simulink model "ES229A_HwTqCorrln"  (R2013b)
settings: Solver=FixedStepDiscrete  SolverMode=SingleTasking  StartTime=0.0  StopTime=1  FixedStep=0.002  RelTol=1e-3
undefined symbols (not defined in the file): ARCHGLBPRM_100MILLISEC_SEC_F32, FLTINJ_HWTQCORRLN_HWTQIDPTSIG, HwTqCorrlnChACmnModCmpLpFilActvnThd, HwTqCorrlnChACmnModCmpLpFilOutpLim, HwTqCorrlnChAImdtCorrlnChkFailThd, HwTqCorrlnChAImdtCorrlnChkPassThd, HwTqCorrlnChAStabStClrFltThd, HwTqCorrlnChAStabStSetFltThd, HwTqCorrlnChATqSumMaxLim, HwTqCorrlnChATraSumClrFltThd, HwTqCorrlnChATraSumSetFltThd, HwTqCorrlnChBCmnModCmpLpFilActvnThd, HwTqCorrlnChBCmnModCmpLpFilOutpLim, HwTqCorrlnChBImdtCorrlnChkFailThd, HwTqCorrlnChBImdtCorrlnChkPassThd, HwTqCorrlnChBStabStClrFltThd, HwTqCorrlnChBStabStSetFltThd, HwTqCorrlnChBTqSumMaxLim, HwTqCorrlnChBTraSumClrFltThd, HwTqCorrlnChBTraSumSetFltThd, HwTqCorrlnMaxStallTqA, HwTqCorrlnMaxStallTqB, HwTqCorrlnMaxStallTqC, HwTqCorrlnMaxStallTqD, HWTQSCA_CNT_U08, NtcNr1, NtcSts1, PARAMETERBYTE_CNT_U08, sigbuilder_block, SigQlfr1, STABSTLPFILSTVARIDELTALIM_HWNWTMTR_F32
libraries: simulink x25, Fil x12, NxtrLim x10, NxtrAbslt x6, FixdToFloat x2, FloatToFixdWithRound x2, LnrIntrpn x2, NxtrNvM x2
(part 2 of 4)

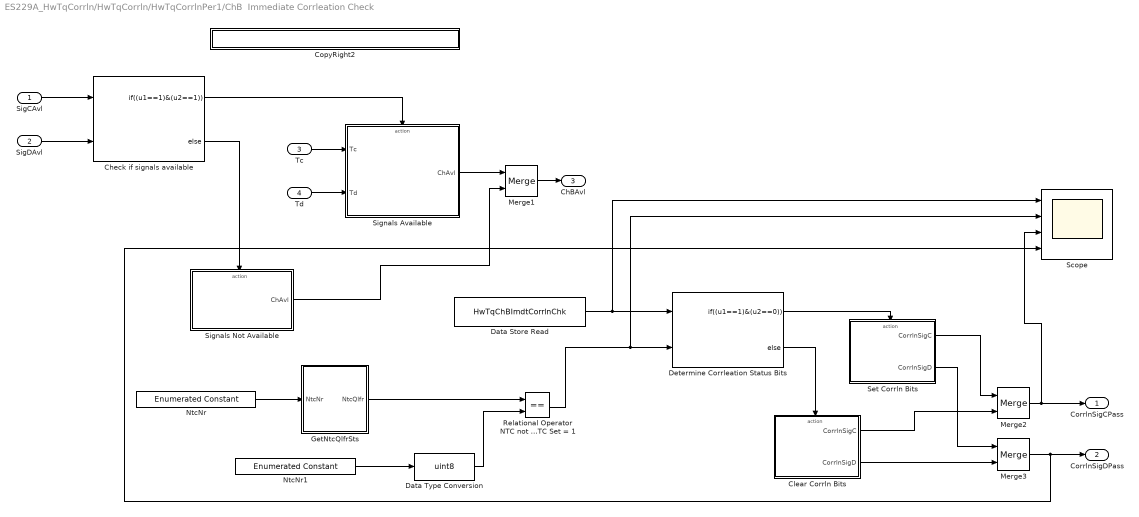
== system ES229A_HwTqCorrln/HwTqCorrln/HwTqCorrlnPer1/ChB  Immediate Corrleation Check ==
  SigCAvl : Inport
  SigDAvl : Inport  Port=2
  Tc : Inport  Port=3
  Td : Inport  Port=4
  Check if signals available : If  NumInputs=2  IfExpression=(u1==1)&(u2==1)
  Clear Corrln Bits : Subsystem  TreatAsAtomicUnit=on
  CopyRight2 : Subsystem  Description=|  mask(Copyright Information){none=on}
      | Copyright info block.                                               
      |                                                                     
      | Place copyright information at the top of every subsystem in design.
      mask prompts: none "No parameters"
      mask help: Place copyright information at the top of every subsystem in design.
      mask Display:
      | NxtrConf = 'Nexteer Confidential';
      | 
      | sys = bdroot; %handle for the current model ("system")
      | first = get_param(sys,'Created');
      | first = first(end-3:end);  %year is last four digits
      | 
      | last = get_param(sys,'LastModifiedDate');
      | if isempty(last)
      |     last = datestr(now,'yyyy');
      | else
      |     last = last(end-3:end);
      | end
      | 
      | if strcmp(first,last)
      |     fprintf('%s -- Copyright %s Nexteer',NxtrConf,first)
      | else
      |     fprintf('%s -- %s%s- %s Nexteer',NxtrConf,char(169),first,last)
      | end
  Data Store Read : DataStoreRead  DataStoreName=HwTqChBImdtCorrlnChk
  Data Type Conversion : DataTypeConversion  OutDataTypeStr=uint8
  Determine Corrleation Status Bits : If  NumInputs=2  IfExpression=(u1==1)&(u2==0)
  GetNtcQlfrSts : Subsystem  RequirementInfo={} %GIDa_b9216dd4_3d01_4ddd_95ef_a4798394f877  TreatAsAtomicUnit=on  mask(GetNTC){}
      mask help: GetNTC library block
      settings: RTWSystemCode=Inline
  Merge1 : Merge
  Merge2 : Merge
  Merge3 : Merge
  NtcNr : simulink/Sources/Enumerated Constant  OutDataTypeStr=Enum: NtcNr1  Value=NtcNr1.NTCNR_0X071  SampleTime=inf
  NtcNr1 : simulink/Sources/Enumerated Constant  OutDataTypeStr=Enum: SigQlfr1  Value=SigQlfr1.SIGQLFR_FAILD  SampleTime=inf
  "Relational Operator NTC not Set = 0, NTC Set = 1" : RelationalOperator  Operator===  OutDataTypeStr=boolean
  Scope : Scope  NumInputPorts=4
      settings: TimeRange=auto  MaxDataPoints=5000  SaveToWorkspace=off  SaveName=ScopeData8  YMin=-5~-5~-5~-5  YMax=5~5~5~5  SampleTime=-1
  Set Corrln Bits : Subsystem  TreatAsAtomicUnit=on
  Signals Available : Subsystem  RequirementInfo={'linktype_rmi_doors' '0000c477 (/ESG Group/FDD Module Requirements/EA4 Specific/ES229A_HwTqCorrln)' '#ES229A_114' 'true' 'REQ:ES229A_114' '' } %GIDa_b18ea54d_339b_4dd7_8965_346bd4b35b88  TreatAsAtomicUnit=on
  Signals Not Available : Subsystem  RequirementInfo={'linktype_rmi_doors' '0000c477 (/ESG Group/FDD Module Requirements/EA4 Specific/ES229A_HwTqCorrln)' '#ES229A_162' 'true' 'REQ:ES229A_162' '' } %GIDa_09088bdc_3033_45ea_8a6e_b545563978f2  TreatAsAtomicUnit=on
  CorrlnSigCPass : Outport
  CorrlnSigDPass : Outport  Port=2
  ChBAvl : Outport  Port=3
  wires:
  Tc/1 -> Signals Available/1(Tc)
  Td/1 -> Signals Available/2(Td)
  Merge3/1 -> Scope/4, CorrlnSigDPass/1
  Determine Corrleation Status Bits/2 -> Clear Corrln Bits/Action
  Determine Corrleation Status Bits/1 -> Set Corrln Bits/Action
  Set Corrln Bits/1(CorrlnSigC) -> Merge2/1
  Clear Corrln Bits/1(CorrlnSigC) -> Merge2/2
  Clear Corrln Bits/2(CorrlnSigD) -> Merge3/2
  NtcNr/1 -> GetNtcQlfrSts/1(NtcNr)
  Data Type Conversion/1 -> "Relational Operator NTC not Set = 0, NTC Set = 1"/2
  GetNtcQlfrSts/1(NtcQlfr) -> "Relational Operator NTC not Set = 0, NTC Set = 1"/1
  "Relational Operator NTC not Set = 0, NTC Set = 1"/1 -> Determine Corrleation Status Bits/2, Scope/2
  Check if signals available/1 -> Signals Available/Action
  Check if signals available/2 -> Signals Not Available/Action
  Data Store Read/1 -> Scope/1, Determine Corrleation Status Bits/1
  SigCAvl/1 -> Check if signals available/1
  SigDAvl/1 -> Check if signals available/2
  Merge2/1 -> Scope/3, CorrlnSigCPass/1
  Set Corrln Bits/2(CorrlnSigD) -> Merge3/1
  NtcNr1/1 -> Data Type Conversion/1
  Merge1/1 -> ChBAvl/1
  Signals Not Available/1(ChAvl) -> Merge1/2
  Signals Available/1(ChAvl) -> Merge1/1

== system ES229A_HwTqCorrln/HwTqCorrln/HwTqCorrlnPer1/CopyRight2 ==

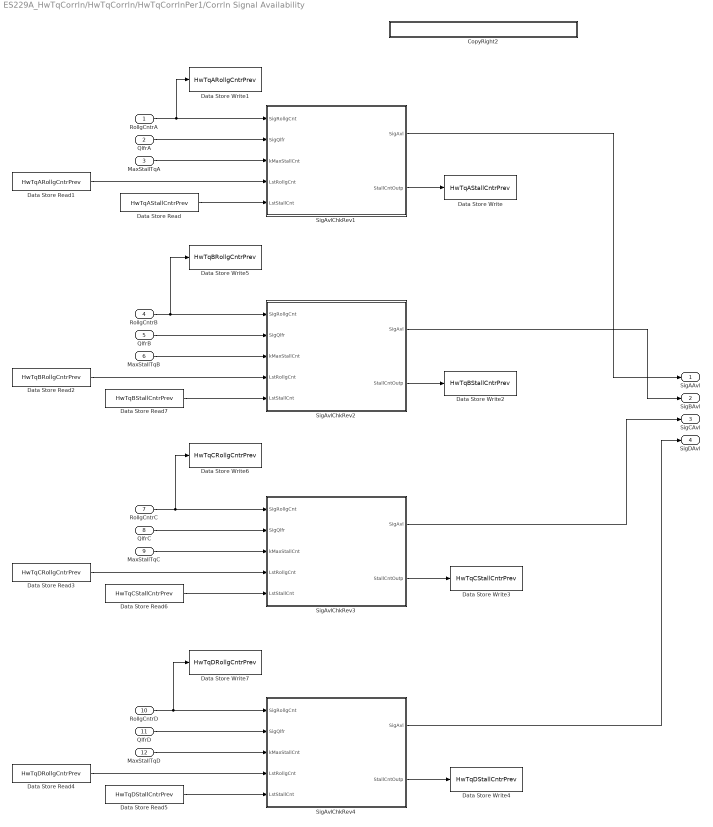
== system ES229A_HwTqCorrln/HwTqCorrln/HwTqCorrlnPer1/Corrln Signal Availability ==
  RollgCntrA : Inport
  QlfrA : Inport  Port=2
  MaxStallTqA : Inport  Port=3
  RollgCntrB : Inport  Port=4
  QlfrB : Inport  Port=5
  MaxStallTqB : Inport  Port=6
  RollgCntrC : Inport  Port=7
  QlfrC : Inport  Port=8
  MaxStallTqC : Inport  Port=9
  RollgCntrD : Inport  Port=10
  QlfrD : Inport  Port=11
  MaxStallTqD : Inport  Port=12
  CopyRight2 : Subsystem  Description=|  mask(Copyright Information){none=on}
      | Copyright info block.                                               
      |                                                                     
      | Place copyright information at the top of every subsystem in design.
      mask prompts: none "No parameters"
      mask help: Place copyright information at the top of every subsystem in design.
      mask Display:
      | NxtrConf = 'Nexteer Confidential';
      | 
      | sys = bdroot; %handle for the current model ("system")
      | first = get_param(sys,'Created');
      | first = first(end-3:end);  %year is last four digits
      | 
      | last = get_param(sys,'LastModifiedDate');
      | if isempty(last)
      |     last = datestr(now,'yyyy');
      | else
      |     last = last(end-3:end);
      | end
      | 
      | if strcmp(first,last)
      |     fprintf('%s -- Copyright %s Nexteer',NxtrConf,first)
      | else
      |     fprintf('%s -- %s%s- %s Nexteer',NxtrConf,char(169),first,last)
      | end
  Data Store Read : DataStoreRead  DataStoreName=HwTqAStallCntrPrev
  Data Store Read1 : DataStoreRead  DataStoreName=HwTqARollgCntrPrev
  Data Store Read2 : DataStoreRead  DataStoreName=HwTqBRollgCntrPrev
  Data Store Read3 : DataStoreRead  DataStoreName=HwTqCRollgCntrPrev
  Data Store Read4 : DataStoreRead  DataStoreName=HwTqDRollgCntrPrev
  Data Store Read5 : DataStoreRead  DataStoreName=HwTqDStallCntrPrev
  Data Store Read6 : DataStoreRead  DataStoreName=HwTqCStallCntrPrev
  Data Store Read7 : DataStoreRead  DataStoreName=HwTqBStallCntrPrev
  Data Store Write : DataStoreWrite  DataStoreName=HwTqAStallCntrPrev
  Data Store Write1 : DataStoreWrite  DataStoreName=HwTqARollgCntrPrev
  Data Store Write2 : DataStoreWrite  DataStoreName=HwTqBStallCntrPrev
  Data Store Write3 : DataStoreWrite  DataStoreName=HwTqCStallCntrPrev
  Data Store Write4 : DataStoreWrite  DataStoreName=HwTqDStallCntrPrev
  Data Store Write5 : DataStoreWrite  DataStoreName=HwTqBRollgCntrPrev
  Data Store Write6 : DataStoreWrite  DataStoreName=HwTqCRollgCntrPrev
  Data Store Write7 : DataStoreWrite  DataStoreName=HwTqDRollgCntrPrev
  SigAvlChkRev1 : Stateflow chart  RequirementInfo="{'linktype_rmi_doors' '0000c477 (/ESG Group/FDD Module Requirements/EA4 Specific/ES229A_HwTqCorrln)' '#ES229A_147' 'true' 'REQ:  ES229A_147' '' } %GIDa_f3ad2930_eb6a_4ba6_add5_8e619e3a87ba"  TreatAsAtomicUnit=on
      settings: PermitHierarchicalResolution=ParametersOnly
  SigAvlChkRev2 : Stateflow chart  RequirementInfo="{'linktype_rmi_doors' '0000c477 (/ESG Group/FDD Module Requirements/EA4 Specific/ES229A_HwTqCorrln)' '#ES229A_148' 'true' 'REQ:  ES229A_148' '' } %GIDa_f0910f57_d48e_4519_bdf9_e92a075f72c3"  TreatAsAtomicUnit=on
      settings: PermitHierarchicalResolution=ParametersOnly
  SigAvlChkRev3 : Stateflow chart  RequirementInfo="{'linktype_rmi_doors' '0000c477 (/ESG Group/FDD Module Requirements/EA4 Specific/ES229A_HwTqCorrln)' '#ES229A_149' 'true' 'REQ:  ES229A_149' '' } %GIDa_0d95f7f7_e61d_4be7_9e90_a8711bbf9663"  TreatAsAtomicUnit=on
      settings: PermitHierarchicalResolution=ParametersOnly
  SigAvlChkRev4 : Stateflow chart  RequirementInfo="{'linktype_rmi_doors' '0000c477 (/ESG Group/FDD Module Requirements/EA4 Specific/ES229A_HwTqCorrln)' '#ES229A_150' 'true' 'REQ:  ES229A_150' '' } %GIDa_ea9f5c51_c346_4ca3_b0d6_fdb5e1bf07d3"  TreatAsAtomicUnit=on
      settings: PermitHierarchicalResolution=ParametersOnly
  SigAAvl : Outport
  SigBAvl : Outport  Port=2
  SigCAvl : Outport  Port=3
  SigDAvl : Outport  Port=4
  wires:
  SigAvlChkRev1/1(SigAvl) -> SigAAvl/1
  SigAvlChkRev2/1(SigAvl) -> SigBAvl/1
  SigAvlChkRev3/1(SigAvl) -> SigCAvl/1
  SigAvlChkRev4/1(SigAvl) -> SigDAvl/1
  RollgCntrA/1 -> Data Store Write1/1, SigAvlChkRev1/1(SigRollgCnt)
  QlfrA/1 -> SigAvlChkRev1/2(SigQlfr)
  MaxStallTqA/1 -> SigAvlChkRev1/3(kMaxStallCnt)
  RollgCntrB/1 -> Data Store Write5/1, SigAvlChkRev2/1(SigRollgCnt)
  QlfrB/1 -> SigAvlChkRev2/2(SigQlfr)
  MaxStallTqB/1 -> SigAvlChkRev2/3(kMaxStallCnt)
  RollgCntrC/1 -> Data Store Write6/1, SigAvlChkRev3/1(SigRollgCnt)
  QlfrC/1 -> SigAvlChkRev3/2(SigQlfr)
  MaxStallTqC/1 -> SigAvlChkRev3/3(kMaxStallCnt)
  RollgCntrD/1 -> Data Store Write7/1, SigAvlChkRev4/1(SigRollgCnt)
  QlfrD/1 -> SigAvlChkRev4/2(SigQlfr)
  MaxStallTqD/1 -> SigAvlChkRev4/3(kMaxStallCnt)
  Data Store Read1/1 -> SigAvlChkRev1/4(LstRollgCnt)
  SigAvlChkRev1/2(StallCntOutp) -> Data Store Write/1
  Data Store Read/1 -> SigAvlChkRev1/5(LstStallCnt)
  Data Store Read2/1 -> SigAvlChkRev2/4(LstRollgCnt)
  SigAvlChkRev2/2(StallCntOutp) -> Data Store Write2/1
  Data Store Read3/1 -> SigAvlChkRev3/4(LstRollgCnt)
  SigAvlChkRev3/2(StallCntOutp) -> Data Store Write3/1
  Data Store Read4/1 -> SigAvlChkRev4/4(LstRollgCnt)
  SigAvlChkRev4/2(StallCntOutp) -> Data Store Write4/1
  Data Store Read5/1 -> SigAvlChkRev4/5(LstStallCnt)
  Data Store Read6/1 -> SigAvlChkRev3/5(LstStallCnt)
  Data Store Read7/1 -> SigAvlChkRev2/5(LstStallCnt)

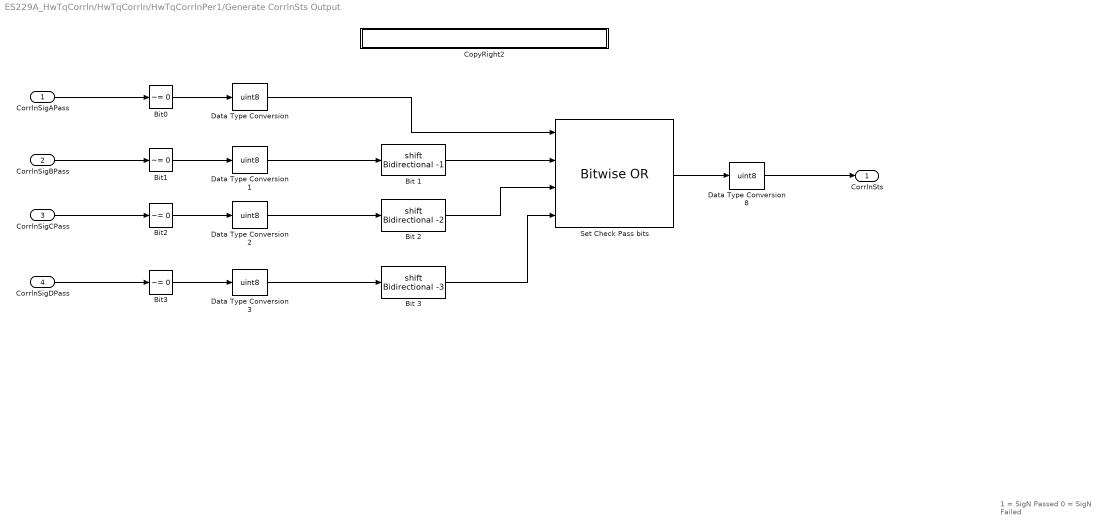
== system ES229A_HwTqCorrln/HwTqCorrln/HwTqCorrlnPer1/Generate CorrlnSts Output ==
  note: 1 = SigN Passed
      | 0 = SigN Failed
  "CorrlnSigAPass " : Inport
  CorrlnSigBPass : Inport  Port=2
  CorrlnSigCPass : Inport  Port=3
  CorrlnSigDPass : Inport  Port=4
  Bit 1 : ArithShift  BitShiftNumber=-1
  Bit 2 : ArithShift  BitShiftNumber=-2
  Bit 3 : ArithShift  BitShiftNumber=-3
  Bit{0..3} (4 alike) : simulink/Logic and Bit Operations/Compare To Zero  relop=~=  OutDataTypeStr=boolean
  CopyRight2 : Subsystem  Description=|  mask(Copyright Information){none=on}
      | Copyright info block.                                               
      |                                                                     
      | Place copyright information at the top of every subsystem in design.
      mask prompts: none "No parameters"
      mask help: Place copyright information at the top of every subsystem in design.
      mask Display:
      | NxtrConf = 'Nexteer Confidential';
      | 
      | sys = bdroot; %handle for the current model ("system")
      | first = get_param(sys,'Created');
      | first = first(end-3:end);  %year is last four digits
      | 
      | last = get_param(sys,'LastModifiedDate');
      | if isempty(last)
      |     last = datestr(now,'yyyy');
      | else
      |     last = last(end-3:end);
      | end
      | 
      | if strcmp(first,last)
      |     fprintf('%s -- Copyright %s Nexteer',NxtrConf,first)
      | else
      |     fprintf('%s -- %s%s- %s Nexteer',NxtrConf,char(169),first,last)
      | end
  Data Type Conversion{,1..3,8} (5 alike) : DataTypeConversion  OutDataTypeStr=uint8
  Set Check Pass bits : simulink/Logic and Bit Operations/Bitwise Operator  logicop=OR  UseBitMask=off  NumInputPorts=4  BitMask=bin2dec('11011001')  BitMaskRealWorld=Stored Integer
  CorrlnSts : Outport
  wires:
  Bit0/1 -> Data Type Conversion/1
  Bit1/1 -> Data Type Conversion1/1
  Bit2/1 -> Data Type Conversion2/1
  Bit3/1 -> Data Type Conversion3/1
  Data Type Conversion1/1 -> Bit 1/1
  Data Type Conversion2/1 -> Bit 2/1
  Data Type Conversion3/1 -> Bit 3/1
  Data Type Conversion/1 -> Set Check Pass bits/1
  Bit 1/1 -> Set Check Pass bits/2
  "CorrlnSigAPass "/1 -> Bit0/1
  CorrlnSigBPass/1 -> Bit1/1
  Set Check Pass bits/1 -> Data Type Conversion8/1
  Data Type Conversion8/1 -> CorrlnSts/1
  CorrlnSigDPass/1 -> Bit3/1
  CorrlnSigCPass/1 -> Bit2/1
  Bit 2/1 -> Set Check Pass bits/3
  Bit 3/1 -> Set Check Pass bits/4

== system ES229A_HwTqCorrln/HwTqCorrln/HwTqCorrlnPer2/ChA Long Term Correlation Fault Determination ==
  In1 : Inport
  In2 : Inport  Port=2
  Ch A Set/Clear Fault : Subsystem  RequirementInfo="{'linktype_rmi_doors' '0000c477 (/ESG Group/FDD Module Requirements/EA4 Specific/ES229A_HwTqCorrln)' '#ES229A_22' 'true' 'REQ:  ES229A_22' '' ; 'linktype_rmi_doors' '0000c477 (/ESG Group/FDD Module Requirements/EA4 Specific/ES229A_HwTqCorrln)' '#ES229A_27' 'true' 'REQ:  ES229A_27' '' ; 'linktype_rmi_doors' '0000c477 (/ESG Group/FDD Module Requirements/EA4 Specific/ES229A_HwTqCorrln)' '#ES229A_30' 'true' 'REQ:  ES229A_30' '' } %GIDa_b0c45f06_e766_43fc_a6ed_3bbbb3b7369d"
  Ch A Variable Fc Transient Fault LPF : Subsystem  RequirementInfo="{'linktype_rmi_doors' '0000c477 (/ESG Group/FDD Module Requirements/EA4 Specific/ES229A_HwTqCorrln)' '#ES229A_117' 'true' 'REQ:  ES229A_117' '' } %GIDa_ea439a28_ceea_4186_9e1d_b468c533a47e"
  ChA CMC LPF Limit : Subsystem  RequirementInfo="{'linktype_rmi_doors' '0000c477 (/ESG Group/FDD Module Requirements/EA4 Specific/ES229A_HwTqCorrln)' '#ES229A_125' 'true' 'REQ:  ES229A_125' '' } %GIDa_8fede557_c77e_4860_a804_3790181f3d16"
  ChA Trq Sum Limit : Subsystem  RequirementInfo="{'linktype_rmi_doors' '0000c477 (/ESG Group/FDD Module Requirements/EA4 Specific/ES229A_HwTqCorrln)' '#ES229A_116' 'true' 'REQ:  ES229A_116' '' } %GIDa_2d7a6ed5_abf9_41fe_9eac_ff6e1e411ede"
  CopyRight2 : Subsystem  Description=|  mask(Copyright Information){none=on}
      | Copyright info block.                                               
      |                                                                     
      | Place copyright information at the top of every subsystem in design.
      mask prompts: none "No parameters"
      mask help: Place copyright information at the top of every subsystem in design.
      mask Display:
      | NxtrConf = 'Nexteer Confidential';
      | 
      | sys = bdroot; %handle for the current model ("system")
      | first = get_param(sys,'Created');
      | first = first(end-3:end);  %year is last four digits
      | 
      | last = get_param(sys,'LastModifiedDate');
      | if isempty(last)
      |     last = datestr(now,'yyyy');
      | else
      |     last = last(end-3:end);
      | end
      | 
      | if strcmp(first,last)
      |     fprintf('%s -- Copyright %s Nexteer',NxtrConf,first)
      | else
      |     fprintf('%s -- %s%s- %s Nexteer',NxtrConf,char(169),first,last)
      | end
  Data Store Read : DataStoreRead  DataStoreName=HwTqChAStabStLpFil  DataStoreElements=HwTqChAStabStLpFil.FilSt
  TqSumLmt : Outport
  HwTqChACorrlnTraErr : Outport  Port=2
  wires:
  ChA Trq Sum Limit/1(Out1) -> Ch A Variable Fc Transient Fault LPF/1(TrqSumLmt), TqSumLmt/1
  Ch A Variable Fc Transient Fault LPF/1(TraLpFilOp) -> Ch A Set/Clear Fault/2(TraLpFilOp)
  Data Store Read/1 -> Ch A Set/Clear Fault/1(StabStFilOutp)
  In1/1 -> ChA Trq Sum Limit/1(In1)
  In2/1 -> ChA Trq Sum Limit/2(In2)
  ChA CMC LPF Limit/1(CmnModCmpLpFilOutpLmt) -> Ch A Set/Clear Fault/3(CMCLpFLimOutp)
  Ch A Set/Clear Fault/1(HwTqChACorrlnTraErr) -> HwTqChACorrlnTraErr/1

== system ES229A_HwTqCorrln/HwTqCorrln/HwTqCorrlnPer2/ChB Long Term Correlation Fault Determination ==
  In1 : Inport
  In2 : Inport  Port=2
  Ch B CMC LPF Limit : Subsystem  RequirementInfo="{'linktype_rmi_doors' '0000c477 (/ESG Group/FDD Module Requirements/EA4 Specific/ES229A_HwTqCorrln)' '#ES229A_135' 'true' 'REQ:  ES229A_135' '' } %GIDa_46d375f2_44d9_4e04_84c6_510bfd0f4870"
  Ch B Set/Clear Fault : Subsystem  RequirementInfo="{'linktype_rmi_doors' '0000c477 (/ESG Group/FDD Module Requirements/EA4 Specific/ES229A_HwTqCorrln)' '#ES229A_90' 'true' 'REQ:  ES229A_90' '' ; 'linktype_rmi_doors' '0000c477 (/ESG Group/FDD Module Requirements/EA4 Specific/ES229A_HwTqCorrln)' '#ES229A_95' 'true' 'REQ:  ES229A_95' '' ; 'linktype_rmi_doors' '0000c477 (/ESG Group/FDD Module Requirements/EA4 Specific/ES229A_HwTqCorrln)' '#ES229A_98' 'true' 'REQ:  ES229A_98' '' } %GIDa_6e3ce5d5_592b_4837_9faf_f2fde9cbfbed"
  Ch B Variable Fc Transient Fault LPF : Subsystem  RequirementInfo="{'linktype_rmi_doors' '0000c477 (/ESG Group/FDD Module Requirements/EA4 Specific/ES229A_HwTqCorrln)' '#ES229A_131' 'true' 'REQ:  ES229A_131' '' } %GIDa_7683c1c9_f66a_4896_85a9_2009ee0ab3a0"
  ChB Trq Sum Limit : Subsystem  RequirementInfo="{'linktype_rmi_doors' '0000c477 (/ESG Group/FDD Module Requirements/EA4 Specific/ES229A_HwTqCorrln)' '#ES229A_130' 'true' 'REQ:  ES229A_130' '' } %GIDa_ba216592_e3df_4c1a_86c0_3647f1bb1480"
  CopyRight2 : Subsystem  Description=|  mask(Copyright Information){none=on}
      | Copyright info block.                                               
      |                                                                     
      | Place copyright information at the top of every subsystem in design.
      mask prompts: none "No parameters"
      mask help: Place copyright information at the top of every subsystem in design.
      mask Display:
      | NxtrConf = 'Nexteer Confidential';
      | 
      | sys = bdroot; %handle for the current model ("system")
      | first = get_param(sys,'Created');
      | first = first(end-3:end);  %year is last four digits
      | 
      | last = get_param(sys,'LastModifiedDate');
      | if isempty(last)
      |     last = datestr(now,'yyyy');
      | else
      |     last = last(end-3:end);
      | end
      | 
      | if strcmp(first,last)
      |     fprintf('%s -- Copyright %s Nexteer',NxtrConf,first)
      | else
      |     fprintf('%s -- %s%s- %s Nexteer',NxtrConf,char(169),first,last)
      | end
  Data Store Read : DataStoreRead  DataStoreName=HwTqChBStabStLpFil  DataStoreElements=HwTqChBStabStLpFil.FilSt
  TqSumLmt : Outport
  HwTqChBCorrlnTraErr : Outport  Port=2
  wires:
  ChB Trq Sum Limit/1(Out1) -> Ch B Variable Fc Transient Fault LPF/1(TrqSumLmt), TqSumLmt/1
  Data Store Read/1 -> Ch B Set/Clear Fault/1(StabStFilOutp)
  In1/1 -> ChB Trq Sum Limit/1(In1)
  In2/1 -> ChB Trq Sum Limit/2(In2)
  Ch B Variable Fc Transient Fault LPF/1(TraLpFilOp) -> Ch B Set/Clear Fault/2(TraLpFilOp)
  Ch B CMC LPF Limit/1(CmnModCmpLpFilOutpLmt) -> Ch B Set/Clear Fault/3(CmnModCmpLpFilOutpLmt)
  Ch B Set/Clear Fault/1(HwTqChBCorrlnTraErr) -> HwTqChBCorrlnTraErr/1

== system ES229A_HwTqCorrln/HwTqCorrln/HwTqCorrlnPer2/CopyRight2 ==

== system ES229A_HwTqCorrln/HwTqCorrln/HwTqCorrlnPer2/FltInj_u08 ==
  note: Inport #2 must be enumeration
      | Enum: FltInjectionLocType
  note: EA4.x Fault Injection
  note: This block requires no modification by FDD author.
      |
      | This block does not actually simulate any fault injection.  It is simply a pass-thru.
      |
      | The Enum port (#2) simply terminates its signal, but we are trying to force the FDD author
      | to properly use the FltInjectionLocType enumeration in FDD model.
  Signal : Inport
  Enum : Inport  Port=2
  Terminator : Terminator
  Out1 : Outport
  wires:
  Enum/1 -> Terminator/1
  Signal/1 -> Out1/1

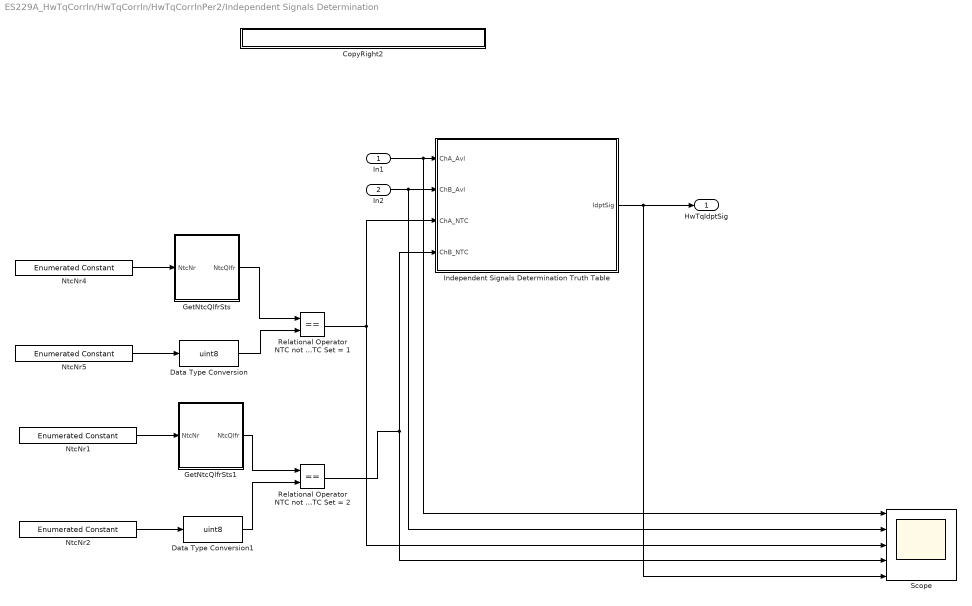
== system ES229A_HwTqCorrln/HwTqCorrln/HwTqCorrlnPer2/Independent Signals Determination ==
  In1 : Inport
  In2 : Inport  Port=2
  CopyRight2 : Subsystem  Description=|  mask(Copyright Information){none=on}
      | Copyright info block.                                               
      |                                                                     
      | Place copyright information at the top of every subsystem in design.
      mask prompts: none "No parameters"
      mask help: Place copyright information at the top of every subsystem in design.
      mask Display:
      | NxtrConf = 'Nexteer Confidential';
      | 
      | sys = bdroot; %handle for the current model ("system")
      | first = get_param(sys,'Created');
      | first = first(end-3:end);  %year is last four digits
      | 
      | last = get_param(sys,'LastModifiedDate');
      | if isempty(last)
      |     last = datestr(now,'yyyy');
      | else
      |     last = last(end-3:end);
      | end
      | 
      | if strcmp(first,last)
      |     fprintf('%s -- Copyright %s Nexteer',NxtrConf,first)
      | else
      |     fprintf('%s -- %s%s- %s Nexteer',NxtrConf,char(169),first,last)
      | end
  Data Type Conversion : DataTypeConversion  OutDataTypeStr=uint8
  Data Type Conversion1 : DataTypeConversion  OutDataTypeStr=uint8
  GetNtcQlfrSts : Subsystem  RequirementInfo={} %GIDa_fb734de9_fb4a_41cf_8ba2_524fea9d7dff  TreatAsAtomicUnit=on  mask(GetNTC){}
      mask help: GetNTC library block
      settings: RTWSystemCode=Inline
  GetNtcQlfrSts1 : Subsystem  RequirementInfo={} %GIDa_5980e2fa_af68_42ea_b5e0_531fab9d926f  TreatAsAtomicUnit=on  mask(GetNTC){}
      mask help: GetNTC library block
      settings: RTWSystemCode=Inline
  Independent Signals Determination Truth Table : Truth Table  TreatAsAtomicUnit=on
      settings: PermitHierarchicalResolution=ParametersOnly
  NtcNr1 : simulink/Sources/Enumerated Constant  OutDataTypeStr=Enum: NtcNr1  Value=NtcNr1.NTCNR_0X071  SampleTime=inf
  NtcNr2 : simulink/Sources/Enumerated Constant  OutDataTypeStr=Enum: SigQlfr1  Value=SigQlfr1.SIGQLFR_FAILD  SampleTime=inf
  NtcNr4 : simulink/Sources/Enumerated Constant  OutDataTypeStr=Enum: NtcNr1  Value=NtcNr1.NTCNR_0X070  SampleTime=inf
  NtcNr5 : simulink/Sources/Enumerated Constant  OutDataTypeStr=Enum: SigQlfr1  Value=SigQlfr1.SIGQLFR_FAILD  SampleTime=inf
  "Relational Operator NTC not Set = 0, NTC Set = 1" : RelationalOperator  Operator===  OutDataTypeStr=boolean
  "Relational Operator NTC not Set = 0, NTC Set = 2" : RelationalOperator  Operator===  OutDataTypeStr=boolean
  Scope : Scope  NumInputPorts=5
      settings: TimeRange=auto  MaxDataPoints=5000  SaveToWorkspace=off  SaveName=ScopeData6  YMin=-5~-5~-5~-5~-5  YMax=5~5~5~5~5  SampleTime=-1
  HwTqIdptSig : Outport
  wires:
  Independent Signals Determination Truth Table/1(IdptSig) -> Scope/5, HwTqIdptSig/1
  "Relational Operator NTC not Set = 0, NTC Set = 1"/1 -> Scope/3, Independent Signals Determination Truth Table/3(ChA_NTC)
  "Relational Operator NTC not Set = 0, NTC Set = 2"/1 -> Independent Signals Determination Truth Table/4(ChB_NTC), Scope/4
  NtcNr4/1 -> GetNtcQlfrSts/1(NtcNr)
  NtcNr5/1 -> Data Type Conversion/1
  GetNtcQlfrSts/1(NtcQlfr) -> "Relational Operator NTC not Set = 0, NTC Set = 1"/1
  Data Type Conversion/1 -> "Relational Operator NTC not Set = 0, NTC Set = 1"/2
  NtcNr1/1 -> GetNtcQlfrSts1/1(NtcNr)
  NtcNr2/1 -> Data Type Conversion1/1
  GetNtcQlfrSts1/1(NtcQlfr) -> "Relational Operator NTC not Set = 0, NTC Set = 2"/1
  Data Type Conversion1/1 -> "Relational Operator NTC not Set = 0, NTC Set = 2"/2
  In1/1 -> Scope/1, Independent Signals Determination Truth Table/1(ChA_Avl)
  In2/1 -> Scope/2, Independent Signals Determination Truth Table/2(ChB_Avl)

== system ES229A_HwTqCorrln/HwTqCorrln/HwTqCorrlnPer3/ChA Long Term Offset Compensation ==
  Hw Tq : Inport
  TqSumLmt : Inport  Port=2
  ChA CMC LPF : Subsystem  RequirementInfo="{'linktype_rmi_doors' '0000c477 (/ESG Group/FDD Module Requirements/EA4 Specific/ES229A_HwTqCorrln)' '#ES229A_123' 'true' 'REQ:  ES229A_123' '' ; 'linktype_rmi_doors' '0000c477 (/ESG Group/FDD Module Requirements/EA4 Specific/ES229A_HwTqCorrln)' '#ES229A_124' 'true' 'REQ:  ES229A_124' '' ; 'linktype_rmi_doors' '0000c477 (/ESG Group/FDD Module Requirements/EA4 Specific/ES229A_HwTqCorrln)' '#ES229A_143' 'true' 'REQ:  ES229A_143' '' } %GIDa_a04721c7_3239_47d5_aea4_3dad886457bb"
  CopyRight1 : Subsystem  Description=|  mask(Copyright Information){none=on}
      | Copyright info block.                                               
      |                                                                     
      | Place copyright information at the top of every subsystem in design.
      mask prompts: none "No parameters"
      mask help: Place copyright information at the top of every subsystem in design.
      mask Display:
      | NxtrConf = 'Nexteer Confidential';
      | 
      | sys = bdroot; %handle for the current model ("system")
      | first = get_param(sys,'Created');
      | first = first(end-3:end);  %year is last four digits
      | 
      | last = get_param(sys,'LastModifiedDate');
      | if isempty(last)
      |     last = datestr(now,'yyyy');
      | else
      |     last = last(end-3:end);
      | end
      | 
      | if strcmp(first,last)
      |     fprintf('%s -- Copyright %s Nexteer',NxtrConf,first)
      | else
      |     fprintf('%s -- %s%s- %s Nexteer',NxtrConf,char(169),first,last)
      | end
  CopyRight2 : Subsystem  Description=|  mask(Copyright Information){none=on}
      | Copyright info block.                                               
      |                                                                     
      | Place copyright information at the top of every subsystem in design.
      mask prompts: none "No parameters"
      mask help: Place copyright information at the top of every subsystem in design.
      mask Display:
      | NxtrConf = 'Nexteer Confidential';
      | 
      | sys = bdroot; %handle for the current model ("system")
      | first = get_param(sys,'Created');
      | first = first(end-3:end);  %year is last four digits
      | 
      | last = get_param(sys,'LastModifiedDate');
      | if isempty(last)
      |     last = datestr(now,'yyyy');
      | else
      |     last = last(end-3:end);
      | end
      | 
      | if strcmp(first,last)
      |     fprintf('%s -- Copyright %s Nexteer',NxtrConf,first)
      | else
      |     fprintf('%s -- %s%s- %s Nexteer',NxtrConf,char(169),first,last)
      | end
  Data Store Write : DataStoreWrite  DataStoreName=HwTqChAStabStLpFil  DataStoreElements=HwTqChAStabStLpFil.FilSt
  FilLpUpdOutp : Fil/FilLpUpdOutp  RequirementInfo="{'linktype_rmi_doors' '0000c477 (/ESG Group/FDD Module Requirements/EA4 Specific/ES229A_HwTqCorrln)' '#ES229A_118' 'true' 'REQ:  ES229A_118' '' } %GIDa_15ab5420_2233_427b_b552_dec1c9208537"  StVar=HwTqChAStabStLpFil
      settings: AttributesFormatString=StVar: %<StVar>
  Limit StabStLPF Output : Subsystem
  wires:
  FilLpUpdOutp/1 -> Limit StabStLPF Output/1(In1)
  TqSumLmt/1 -> FilLpUpdOutp/1, ChA CMC LPF/2(TqSumLmt)
  Hw Tq/1 -> ChA CMC LPF/1(In1)
  Limit StabStLPF Output/1(Out1) -> Data Store Write/1

== system ES229A_HwTqCorrln/HwTqCorrln/HwTqCorrlnPer3/ChB Long Term Offset Compensation ==
  Hw Tq : Inport
  TqSumLmt : Inport  Port=2
  ChB CMC LPF : Subsystem  RequirementInfo="{'linktype_rmi_doors' '0000c477 (/ESG Group/FDD Module Requirements/EA4 Specific/ES229A_HwTqCorrln)' '#ES229A_133' 'true' 'REQ:  ES229A_133' '' ; 'linktype_rmi_doors' '0000c477 (/ESG Group/FDD Module Requirements/EA4 Specific/ES229A_HwTqCorrln)' '#ES229A_134' 'true' 'REQ:  ES229A_134' '' ; 'linktype_rmi_doors' '0000c477 (/ESG Group/FDD Module Requirements/EA4 Specific/ES229A_HwTqCorrln)' '#ES229A_155' 'true' 'REQ:  ES229A_155' '' } %GIDa_8ab0b66a_8133_4559_b381_2bcc9397804e"
  CopyRight2 : Subsystem  Description=|  mask(Copyright Information){none=on}
      | Copyright info block.                                               
      |                                                                     
      | Place copyright information at the top of every subsystem in design.
      mask prompts: none "No parameters"
      mask help: Place copyright information at the top of every subsystem in design.
      mask Display:
      | NxtrConf = 'Nexteer Confidential';
      | 
      | sys = bdroot; %handle for the current model ("system")
      | first = get_param(sys,'Created');
      | first = first(end-3:end);  %year is last four digits
      | 
      | last = get_param(sys,'LastModifiedDate');
      | if isempty(last)
      |     last = datestr(now,'yyyy');
      | else
      |     last = last(end-3:end);
      | end
      | 
      | if strcmp(first,last)
      |     fprintf('%s -- Copyright %s Nexteer',NxtrConf,first)
      | else
      |     fprintf('%s -- %s%s- %s Nexteer',NxtrConf,char(169),first,last)
      | end
  Data Store Write : DataStoreWrite  DataStoreName=HwTqChBStabStLpFil  DataStoreElements=HwTqChBStabStLpFil.FilSt
  FilLpUpdOutp : Fil/FilLpUpdOutp  RequirementInfo="{'linktype_rmi_doors' '0000c477 (/ESG Group/FDD Module Requirements/EA4 Specific/ES229A_HwTqCorrln)' '#ES229A_132' 'true' 'REQ:  ES229A_132' '' } %GIDa_31acfed8_fe9d_42a3_839d_28327d6eeb60"  StVar=HwTqChBStabStLpFil
      settings: AttributesFormatString=StVar: %<StVar>
  Limit StabStLPF Output : Subsystem
  wires:
  TqSumLmt/1 -> FilLpUpdOutp/1, ChB CMC LPF/2(In2)
  FilLpUpdOutp/1 -> Limit StabStLPF Output/1(In1)
  Hw Tq/1 -> ChB CMC LPF/1(In1)
  Limit StabStLPF Output/1(Out1) -> Data Store Write/1

== system ES229A_HwTqCorrln/HwTqCorrln/HwTqCorrlnPer3/CopyRight2 ==

== system ES229A_HwTqCorrln/HwTqCorrln/HwTqCorrlnInit1/ChA Common Mode Compensation LPF Init/CopyRight2 ==

== system ES229A_HwTqCorrln/HwTqCorrln/HwTqCorrlnInit1/ChA Transient Fault LPF Init/CopyRight2 ==

== system ES229A_HwTqCorrln/HwTqCorrln/HwTqCorrlnInit1/ChB Common Mode Compensation LPF Init/CopyRight2 ==

== system ES229A_HwTqCorrln/HwTqCorrln/HwTqCorrlnInit1/ChB Transient Fault LPF Init/CopyRight2 ==

== system ES229A_HwTqCorrln/HwTqCorrln/HwTqCorrlnPer1/ChA  Immediate Corrleation Check /Clear Corrln Bits ==
  Action Port : ActionPort  ActionType=else
  Constant : Constant  Value=0  OutDataTypeStr=boolean
  Constant1 : Constant  Value=0  OutDataTypeStr=boolean
  CopyRight2 : Subsystem  Description=|  mask(Copyright Information){none=on}
      | Copyright info block.                                               
      |                                                                     
      | Place copyright information at the top of every subsystem in design.
      mask prompts: none "No parameters"
      mask help: Place copyright information at the top of every subsystem in design.
      mask Display:
      | NxtrConf = 'Nexteer Confidential';
      | 
      | sys = bdroot; %handle for the current model ("system")
      | first = get_param(sys,'Created');
      | first = first(end-3:end);  %year is last four digits
      | 
      | last = get_param(sys,'LastModifiedDate');
      | if isempty(last)
      |     last = datestr(now,'yyyy');
      | else
      |     last = last(end-3:end);
      | end
      | 
      | if strcmp(first,last)
      |     fprintf('%s -- Copyright %s Nexteer',NxtrConf,first)
      | else
      |     fprintf('%s -- %s%s- %s Nexteer',NxtrConf,char(169),first,last)
      | end
  CorrlnSigA : Outport
  CorrlnSigB : Outport  Port=2
  wires:
  Constant1/1 -> CorrlnSigB/1
  Constant/1 -> CorrlnSigA/1

== system ES229A_HwTqCorrln/HwTqCorrln/HwTqCorrlnPer1/ChA  Immediate Corrleation Check /CopyRight2 ==

== system ES229A_HwTqCorrln/HwTqCorrln/HwTqCorrlnPer1/ChA  Immediate Corrleation Check /GetNtcQlfrSts ==
  NtcNr : Inport
  CopyRight2 : Subsystem  Description=|  mask(Copyright Information){none=on}
      | Copyright info block.                                               
      |                                                                     
      | Place copyright information at the top of every subsystem in design.
      mask prompts: none "No parameters"
      mask help: Place copyright information at the top of every subsystem in design.
      mask Display:
      | NxtrConf = 'Nexteer Confidential';
      | 
      | sys = bdroot; %handle for the current model ("system")
      | first = get_param(sys,'Created');
      | first = first(end-3:end);  %year is last four digits
      | 
      | last = get_param(sys,'LastModifiedDate');
      | if isempty(last)
      |     last = datestr(now,'yyyy');
      | else
      |     last = last(end-3:end);
      | end
      | 
      | if strcmp(first,last)
      |     fprintf('%s -- Copyright %s Nexteer',NxtrConf,first)
      | else
      |     fprintf('%s -- %s%s- %s Nexteer',NxtrConf,char(169),first,last)
      | end
  Data Store Read : DataStoreRead  DataStoreName=NtcQlfr0x70
  Terminator : Terminator
  NtcQlfr : Outport
  wires:
  NtcNr/1 -> Terminator/1
  Data Store Read/1 -> NtcQlfr/1

== system ES229A_HwTqCorrln/HwTqCorrln/HwTqCorrlnPer1/ChA  Immediate Corrleation Check /Set Corrln Bits ==
  Action Port : ActionPort  ActionType=then
  Constant : Constant  OutDataTypeStr=boolean
  Constant1 : Constant  OutDataTypeStr=boolean
  CopyRight2 : Subsystem  Description=|  mask(Copyright Information){none=on}
      | Copyright info block.                                               
      |                                                                     
      | Place copyright information at the top of every subsystem in design.
      mask prompts: none "No parameters"
      mask help: Place copyright information at the top of every subsystem in design.
      mask Display:
      | NxtrConf = 'Nexteer Confidential';
      | 
      | sys = bdroot; %handle for the current model ("system")
      | first = get_param(sys,'Created');
      | first = first(end-3:end);  %year is last four digits
      | 
      | last = get_param(sys,'LastModifiedDate');
      | if isempty(last)
      |     last = datestr(now,'yyyy');
      | else
      |     last = last(end-3:end);
      | end
      | 
      | if strcmp(first,last)
      |     fprintf('%s -- Copyright %s Nexteer',NxtrConf,first)
      | else
      |     fprintf('%s -- %s%s- %s Nexteer',NxtrConf,char(169),first,last)
      | end
  CorrlnSigA : Outport
  CorrlnSigB : Outport  Port=2
  wires:
  Constant/1 -> CorrlnSigA/1
  Constant1/1 -> CorrlnSigB/1

== system ES229A_HwTqCorrln/HwTqCorrln/HwTqCorrlnPer1/ChA  Immediate Corrleation Check /Signals Available ==
  Ta : Inport
  Tb : Inport  Port=2
  Action Port : ActionPort  ActionType=then
  Abs : Abs
  Constant : Constant  Value=HWTQSCA_CNT_U08
  Constant1 : Constant  OutDataTypeStr=boolean
  Constant2 : Constant  Value=HwTqCorrlnChAImdtCorrlnChkFailThd
  Constant3 : Constant  Value=HwTqCorrlnChAImdtCorrlnChkPassThd
  CopyRight2 : Subsystem  Description=|  mask(Copyright Information){none=on}
      | Copyright info block.                                               
      |                                                                     
      | Place copyright information at the top of every subsystem in design.
      mask prompts: none "No parameters"
      mask help: Place copyright information at the top of every subsystem in design.
      mask Display:
      | NxtrConf = 'Nexteer Confidential';
      | 
      | sys = bdroot; %handle for the current model ("system")
      | first = get_param(sys,'Created');
      | first = first(end-3:end);  %year is last four digits
      | 
      | last = get_param(sys,'LastModifiedDate');
      | if isempty(last)
      |     last = datestr(now,'yyyy');
      | else
      |     last = last(end-3:end);
      | end
      | 
      | if strcmp(first,last)
      |     fprintf('%s -- Copyright %s Nexteer',NxtrConf,first)
      | else
      |     fprintf('%s -- %s%s- %s Nexteer',NxtrConf,char(169),first,last)
      | end
  Divide : Product  Inputs=*/
  Hold last value : Subsystem  TreatAsAtomicUnit=on
  If1 : If  NumInputs=3  IfExpression=u1>=u2  ElseIfExpressions=u1<=u3
  Imdt Corrln Chk Failed : Subsystem  TreatAsAtomicUnit=on
  Imdt Corrln Chk Passed : Subsystem  TreatAsAtomicUnit=on
  Sum : Sum  Inputs=+|-
  ChAvl : Outport
  wires:
  Constant2/1 -> If1/2
  Abs/1 -> If1/1
  Ta/1 -> Sum/1
  Tb/1 -> Sum/2
  Sum/1 -> Divide/1
  Divide/1 -> Abs/1  "TrqSum"
  Constant/1 -> Divide/2
  Constant3/1 -> If1/3
  If1/1 -> Imdt Corrln Chk Failed/Action
  If1/2 -> Imdt Corrln Chk Passed/Action
  If1/3 -> Hold last value/Action
  Constant1/1 -> ChAvl/1

== system ES229A_HwTqCorrln/HwTqCorrln/HwTqCorrlnPer1/ChA  Immediate Corrleation Check /Signals Not Available ==
  Action Port : ActionPort  ActionType=else
  Constant1 : Constant  Value=0  OutDataTypeStr=boolean
  Constant2 : Constant  Value=0  OutDataTypeStr=boolean
  CopyRight2 : Subsystem  Description=|  mask(Copyright Information){none=on}
      | Copyright info block.                                               
      |                                                                     
      | Place copyright information at the top of every subsystem in design.
      mask prompts: none "No parameters"
      mask help: Place copyright information at the top of every subsystem in design.
      mask Display:
      | NxtrConf = 'Nexteer Confidential';
      | 
      | sys = bdroot; %handle for the current model ("system")
      | first = get_param(sys,'Created');
      | first = first(end-3:end);  %year is last four digits
      | 
      | last = get_param(sys,'LastModifiedDate');
      | if isempty(last)
      |     last = datestr(now,'yyyy');
      | else
      |     last = last(end-3:end);
      | end
      | 
      | if strcmp(first,last)
      |     fprintf('%s -- Copyright %s Nexteer',NxtrConf,first)
      | else
      |     fprintf('%s -- %s%s- %s Nexteer',NxtrConf,char(169),first,last)
      | end
  Data Store Write : DataStoreWrite  DataStoreName=HwTqChAImdtCorrlnChk
  ChAvl : Outport
  wires:
  Constant1/1 -> Data Store Write/1
  Constant2/1 -> ChAvl/1

== system ES229A_HwTqCorrln/HwTqCorrln/HwTqCorrlnPer1/ChB  Immediate Corrleation Check/Clear Corrln Bits ==
  Action Port : ActionPort  ActionType=else
  Constant : Constant  Value=0  OutDataTypeStr=boolean
  Constant1 : Constant  Value=0  OutDataTypeStr=boolean
  CopyRight2 : Subsystem  Description=|  mask(Copyright Information){none=on}
      | Copyright info block.                                               
      |                                                                     
      | Place copyright information at the top of every subsystem in design.
      mask prompts: none "No parameters"
      mask help: Place copyright information at the top of every subsystem in design.
      mask Display:
      | NxtrConf = 'Nexteer Confidential';
      | 
      | sys = bdroot; %handle for the current model ("system")
      | first = get_param(sys,'Created');
      | first = first(end-3:end);  %year is last four digits
      | 
      | last = get_param(sys,'LastModifiedDate');
      | if isempty(last)
      |     last = datestr(now,'yyyy');
      | else
      |     last = last(end-3:end);
      | end
      | 
      | if strcmp(first,last)
      |     fprintf('%s -- Copyright %s Nexteer',NxtrConf,first)
      | else
      |     fprintf('%s -- %s%s- %s Nexteer',NxtrConf,char(169),first,last)
      | end
  CorrlnSigC : Outport
  CorrlnSigD : Outport  Port=2
  wires:
  Constant1/1 -> CorrlnSigD/1
  Constant/1 -> CorrlnSigC/1

== system ES229A_HwTqCorrln/HwTqCorrln/HwTqCorrlnPer1/ChB  Immediate Corrleation Check/CopyRight2 ==

== system ES229A_HwTqCorrln/HwTqCorrln/HwTqCorrlnPer1/ChB  Immediate Corrleation Check/GetNtcQlfrSts ==
  NtcNr : Inport
  CopyRight2 : Subsystem  Description=|  mask(Copyright Information){none=on}
      | Copyright info block.                                               
      |                                                                     
      | Place copyright information at the top of every subsystem in design.
      mask prompts: none "No parameters"
      mask help: Place copyright information at the top of every subsystem in design.
      mask Display:
      | NxtrConf = 'Nexteer Confidential';
      | 
      | sys = bdroot; %handle for the current model ("system")
      | first = get_param(sys,'Created');
      | first = first(end-3:end);  %year is last four digits
      | 
      | last = get_param(sys,'LastModifiedDate');
      | if isempty(last)
      |     last = datestr(now,'yyyy');
      | else
      |     last = last(end-3:end);
      | end
      | 
      | if strcmp(first,last)
      |     fprintf('%s -- Copyright %s Nexteer',NxtrConf,first)
      | else
      |     fprintf('%s -- %s%s- %s Nexteer',NxtrConf,char(169),first,last)
      | end
  Data Store Read : DataStoreRead  DataStoreName=NtcQlfr
  Terminator : Terminator
  NtcQlfr : Outport
  wires:
  NtcNr/1 -> Terminator/1
  Data Store Read/1 -> NtcQlfr/1

== system ES229A_HwTqCorrln/HwTqCorrln/HwTqCorrlnPer1/ChB  Immediate Corrleation Check/Set Corrln Bits ==
  Action Port : ActionPort  ActionType=then
  Constant : Constant  OutDataTypeStr=boolean
  Constant1 : Constant  OutDataTypeStr=boolean
  CopyRight2 : Subsystem  Description=|  mask(Copyright Information){none=on}
      | Copyright info block.                                               
      |                                                                     
      | Place copyright information at the top of every subsystem in design.
      mask prompts: none "No parameters"
      mask help: Place copyright information at the top of every subsystem in design.
      mask Display:
      | NxtrConf = 'Nexteer Confidential';
      | 
      | sys = bdroot; %handle for the current model ("system")
      | first = get_param(sys,'Created');
      | first = first(end-3:end);  %year is last four digits
      | 
      | last = get_param(sys,'LastModifiedDate');
      | if isempty(last)
      |     last = datestr(now,'yyyy');
      | else
      |     last = last(end-3:end);
      | end
      | 
      | if strcmp(first,last)
      |     fprintf('%s -- Copyright %s Nexteer',NxtrConf,first)
      | else
      |     fprintf('%s -- %s%s- %s Nexteer',NxtrConf,char(169),first,last)
      | end
  CorrlnSigC : Outport
  CorrlnSigD : Outport  Port=2
  wires:
  Constant/1 -> CorrlnSigC/1
  Constant1/1 -> CorrlnSigD/1

== system ES229A_HwTqCorrln/HwTqCorrln/HwTqCorrlnPer1/ChB  Immediate Corrleation Check/Signals Available ==
  Tc : Inport
  Td : Inport  Port=2
  Action Port : ActionPort  ActionType=then
  Abs : Abs
  Constant : Constant  Value=HWTQSCA_CNT_U08
  Constant1 : Constant  OutDataTypeStr=boolean
  Constant2 : Constant  Value=HwTqCorrlnChBImdtCorrlnChkFailThd
  Constant3 : Constant  Value=HwTqCorrlnChBImdtCorrlnChkPassThd
  CopyRight2 : Subsystem  Description=|  mask(Copyright Information){none=on}
      | Copyright info block.                                               
      |                                                                     
      | Place copyright information at the top of every subsystem in design.
      mask prompts: none "No parameters"
      mask help: Place copyright information at the top of every subsystem in design.
      mask Display:
      | NxtrConf = 'Nexteer Confidential';
      | 
      | sys = bdroot; %handle for the current model ("system")
      | first = get_param(sys,'Created');
      | first = first(end-3:end);  %year is last four digits
      | 
      | last = get_param(sys,'LastModifiedDate');
      | if isempty(last)
      |     last = datestr(now,'yyyy');
      | else
      |     last = last(end-3:end);
      | end
      | 
      | if strcmp(first,last)
      |     fprintf('%s -- Copyright %s Nexteer',NxtrConf,first)
      | else
      |     fprintf('%s -- %s%s- %s Nexteer',NxtrConf,char(169),first,last)
      | end
  Divide : Product  Inputs=*/
  Hold last value : Subsystem  TreatAsAtomicUnit=on
  If1 : If  NumInputs=3  IfExpression=u1>=u2  ElseIfExpressions=u1<=u3
  Imdt Corrln Chk Failed : Subsystem  TreatAsAtomicUnit=on
  Imdt Corrln Chk Passed : Subsystem  TreatAsAtomicUnit=on
  Sum : Sum  Inputs=+|-
  ChAvl : Outport
  wires:
  Abs/1 -> If1/1
  Tc/1 -> Sum/1
  Td/1 -> Sum/2
  Sum/1 -> Divide/1
  Divide/1 -> Abs/1  "TrqSum"
  Constant/1 -> Divide/2
  Constant2/1 -> If1/2
  Constant3/1 -> If1/3
  If1/2 -> Imdt Corrln Chk Passed/Action
  If1/3 -> Hold last value/Action
  If1/1 -> Imdt Corrln Chk Failed/Action
  Constant1/1 -> ChAvl/1

== system ES229A_HwTqCorrln/HwTqCorrln/HwTqCorrlnPer1/ChB  Immediate Corrleation Check/Signals Not Available ==
  Action Port : ActionPort  ActionType=else
  Constant : Constant  Value=0  OutDataTypeStr=boolean
  Constant1 : Constant  Value=0  OutDataTypeStr=boolean
  CopyRight2 : Subsystem  Description=|  mask(Copyright Information){none=on}
      | Copyright info block.                                               
      |                                                                     
      | Place copyright information at the top of every subsystem in design.
      mask prompts: none "No parameters"
      mask help: Place copyright information at the top of every subsystem in design.
      mask Display:
      | NxtrConf = 'Nexteer Confidential';
      | 
      | sys = bdroot; %handle for the current model ("system")
      | first = get_param(sys,'Created');
      | first = first(end-3:end);  %year is last four digits
      | 
      | last = get_param(sys,'LastModifiedDate');
      | if isempty(last)
      |     last = datestr(now,'yyyy');
      | else
      |     last = last(end-3:end);
      | end
      | 
      | if strcmp(first,last)
      |     fprintf('%s -- Copyright %s Nexteer',NxtrConf,first)
      | else
      |     fprintf('%s -- %s%s- %s Nexteer',NxtrConf,char(169),first,last)
      | end
  Data Store Write : DataStoreWrite  DataStoreName=HwTqChBImdtCorrlnChk
  ChAvl : Outport
  wires:
  Constant/1 -> Data Store Write/1
  Constant1/1 -> ChAvl/1

== system ES229A_HwTqCorrln/HwTqCorrln/HwTqCorrlnPer1/Corrln Signal Availability/CopyRight2 ==

== system ES229A_HwTqCorrln/HwTqCorrln/HwTqCorrlnPer1/Generate CorrlnSts Output/CopyRight2 ==
